simulink subsystem "s0318_alpha_theta_controller_LQR"  (R2019b)
settings: Solver=VariableStepAuto  StartTime=0.0  StopTime=10.0  RelTol=1e-3
model mask{p1=0, p2=0, p3=0, wc=0, cz_ratio=0, pc_ratio=0}
  mask prompts: p1 "Position 1st pole"; p2 "Position 2nd pole"; p3 "Position 3rd pole"; wc "PID cutting frequency"; cz_ratio "PID cutting/zeros ratio"; pc_ratio "PID pole/cutting ratio"
undefined symbols (not defined in the file): K, PARAMS
libraries: simulink x2
settings Model: Creator=francescoceresetti  LastModifiedBy=francescoceresetti

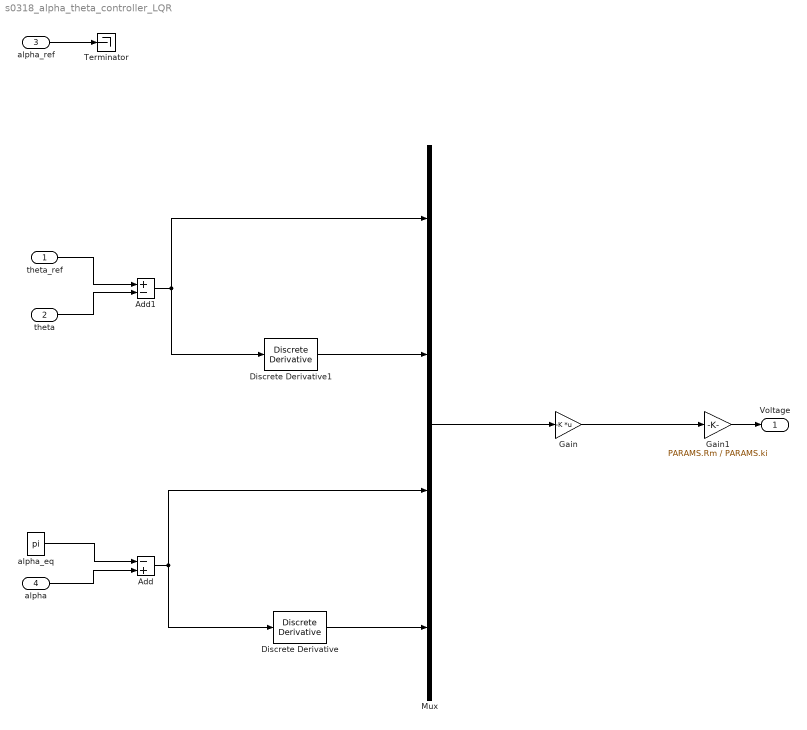
== system s0318_alpha_theta_controller_LQR ==
  theta_ref : Inport
  theta : Inport  Port=2
  alpha_ref : Inport  Port=3
  alpha : Inport  Port=4
  Add : Sum  Inputs=-+
  Add1 : Sum  Inputs=+-
  Discrete Derivative : simulink/Discrete/Discrete Derivative  gainval=1.0  ICPrevScaledInput=pi  OutMin=[]  OutMax=[]  OutDataType=fixdt(1, 16)  OutScaling=2^-10  DoSatur=off
  Discrete Derivative1 : simulink/Discrete/Discrete Derivative  gainval=1.0  ICPrevScaledInput=pi  OutMin=[]  OutMax=[]  OutDataType=fixdt(1, 16)  OutScaling=2^-10  DoSatur=off
  Gain : Gain  Gain=-K  Multiplication=Matrix(K*u)
  Gain1 : Gain  Gain=PARAMS.Rm / PARAMS.ki
  Mux : Mux
  Terminator : Terminator
  "alpha_eq " : Constant  Value=pi
  Voltage : Outport
  wires:
  theta_ref/1 -> Add1/1
  theta/1 -> Add1/2
  alpha_ref/1 -> Terminator/1
  alpha/1 -> Add/2
  "alpha_eq "/1 -> Add/1
  Add/1 -> Discrete Derivative/1, Mux/3
  Discrete Derivative/1 -> Mux/4
  Gain1/1 -> Voltage/1
  Discrete Derivative1/1 -> Mux/2
  Add1/1 -> Mux/1, Discrete Derivative1/1
  Mux/1 -> Gain/1
  Gain/1 -> Gain1/1
